simulink model "sl_ex1"  (R2014a)
settings: Solver=ode45  StartTime=0.0  StopTime=10.0  RelTol=1e-3
settings Model: Creator=liang  LastModifiedBy=liang

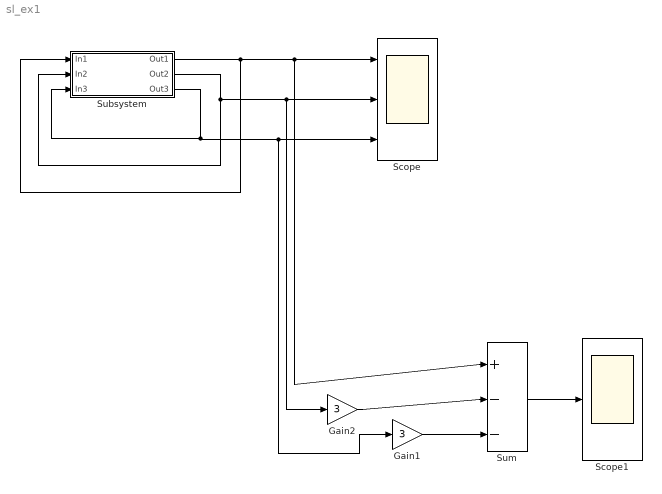
== system sl_ex1 ==
  Gain1 : Gain  Gain=3
  Gain2 : Gain  Gain=3
  Scope : Scope  NumInputPorts=3
      settings: YMin=-5~-5~-5  YMax=5~5~5
  Scope1 : Scope
  Subsystem : Subsystem
  Sum : Sum  Inputs=|+--
  wires:
  Subsystem/1(Out1) -> Sum/1, Scope/1, Subsystem/1(In1)
  Subsystem/3(Out3) -> Gain1/1, Scope/3, Subsystem/3(In3)
  Sum/1 -> Scope1/1
  Subsystem/2(Out2) -> Gain2/1, Scope/2, Subsystem/2(In2)
  Gain2/1 -> Sum/2
  Gain1/1 -> Sum/3

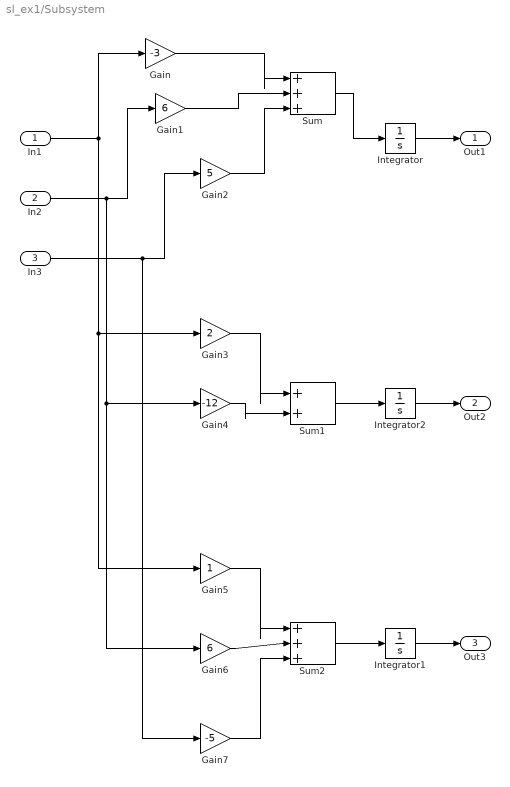
== system sl_ex1/Subsystem ==
  In1 : Inport
  In2 : Inport  Port=2
  In3 : Inport  Port=3
  Gain : Gain  Gain=-3
  Gain1 : Gain  Gain=6
  Gain2 : Gain  Gain=5
  Gain3 : Gain  Gain=2
  Gain4 : Gain  Gain=-12
  Gain5 : Gain
  Gain6 : Gain  Gain=6
  Gain7 : Gain  Gain=-5
  Integrator : Integrator  InitialCondition=1
  Integrator1 : Integrator
  Integrator2 : Integrator
  Sum : Sum  Inputs=|+++
  Sum1 : Sum  Inputs=|++
  Sum2 : Sum  Inputs=|+++
  Out1 : Outport
  Out2 : Outport  Port=2
  Out3 : Outport  Port=3
  wires:
  Integrator/1 -> Out1/1
  Integrator2/1 -> Out2/1
  Integrator1/1 -> Out3/1
  Sum/1 -> Integrator/1
  In1/1 -> Gain5/1, Gain3/1, Gain/1
  Gain/1 -> Sum/1
  In2/1 -> Gain6/1, Gain4/1, Gain1/1
  Gain1/1 -> Sum/2
  In3/1 -> Gain7/1, Gain2/1
  Gain2/1 -> Sum/3
  Sum1/1 -> Integrator2/1
  Gain3/1 -> Sum1/1
  Gain4/1 -> Sum1/2
  Gain5/1 -> Sum2/1
  Gain6/1 -> Sum2/2
  Gain7/1 -> Sum2/3
  Sum2/1 -> Integrator1/1
